simulink model "dimen"  (R2013a)
settings: Solver=ode23tb  StartTime=0.0  StopTime=10.0  RelTol=1e-4
values from neighbouring files (symbols this model uses):
  Cf = 1e-3    (= 0.001)    [dimensionamento.m]
  D0 = 50    [dimensionamento.m]
  DF = 100    [dimensionamento.m]
  ftr = 10e3    (= 10000)    [dimensionamento.m]
  J = 2.22e-2    (= 0.0222)    [dimensionamento.m]
  kt = kt1    [dimensionamento.m]
  La = 28e-3    (= 0.028)    [dimensionamento.m]
  Ra = 2.58    [dimensionamento.m]
  Vsource = Vnom    (= 240)    [dimensionamento.m]
libraries: powerlib x9, simulink x2
settings Model: Creator=dello  LastModifiedBy=dello
settings SolverCC: SolverResetMethod=Robust
settings DataIOCC: SignalLoggingSaveFormat=ModelDataLogs  SignalLoggingName=results

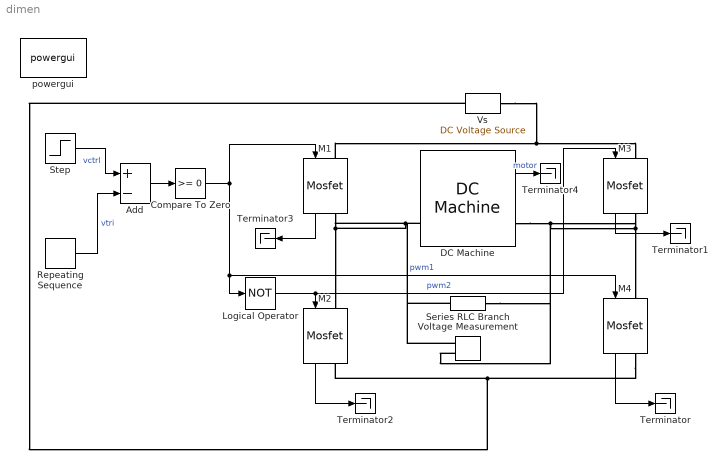
== system dimen ==
  Add : Sum  Inputs=+-
  Compare To Zero : simulink/Logic and Bit Operations/Compare To Zero  relop=>=  OutDataTypeStr=boolean
  DC Machine : powerlib/Machines/DC Machine  PresetModel=No  MechanicalLoad=Torque TL  FieldType=Permanent magnet  ShowDetailedParameters=on  RLa=[ Ra La]  RLf="[ 240  120]"  Laf=1.8  MachineConstant=Torque constant (N.m/A)  Ke=1.8  Kt=kt  J=J  Bm=B  Tf=0  w0=0  Ifinit=1  TsPowergui=0  TsBlock=-1
  Logical Operator : Logic  Operator=NOT  IconShape=distinctive  AllPortsSameDT=off  OutDataTypeStr=boolean
  M{1..4} (4 alike) : powerlib/Power Electronics/Mosfet  Ron=0.1  Lon=0  Rd=0.01  Vfd=0  IC=0  Rs=1e5  Cs=inf  Measurements=on
  Repeating Sequence : simulink/Sources/Repeating Sequence  rep_seq_t=[0 1/ftr/2 1/ftr]  rep_seq_y=[0 100 0]
  Series RLC Branch : powerlib/Elements/Series RLC Branch  LConnTagsString=__new0  RConnTagsString=__new0  BranchType=C  Resistance=1  Inductance=1e-3  SetiL0=off  InitialCurrent=0  Capacitance=Cf  Setx0=off  InitialVoltage=0  Measurements=None
  Step : Step  Before=D0  After=DF  SampleTime=0
  Terminator{,1..4} (5 alike) : Terminator
  Voltage Measurement : powerlib/Measurements/Voltage Measurement  PhasorSimulation=off  OutputType=Complex  PSBequivalent=0
  Vs : powerlib/Electrical Sources/DC Voltage Source  Amplitude=Vsource  Measurements=None
  powergui : powerlib/powergui  Priority=1  SimulationMode=Continuous  SolverType=Tustin  SampleTime=50e-6  frequency=60  SPID=off  DisableSnubberDevices=off  DisableRonSwitches=off  DisableVfSwitches=off  SwTol=0  Interpol=off  DisplayEquations=off  frequencyindice=0  Pbase=100e6  ErrMax=1e-4  Iterations=50  UnitsV=kV  UnitsW=MW  FunctionMessages=off  echomessages=off  HookPort=off  EnableUseOfTLC=off  x0status=blocks  RestoreLinks=warning  ResistiveCurrentMeasurement=off  Frange=[0:2:500]  Ylog=off  Xlog=on  ShowGrid=off  save=off  variable=ZData  ZoomFFT=off  StartTime=0.0  cycles=1  DisplayStyle=1  fundamental=60  FreqAxis=off  MaxFrequency=1000  frequencyindicesteady=1  RmsSteady=1  display=off  Ts=0  methode=off
  wires:
  Logical Operator/1 -> M2/1, M3/1  "pwm2"
  Compare To Zero/1 -> M1/1, M4/1, Logical Operator/1  "pwm1"
  Step/1 -> Add/1  "vctrl"
  Repeating Sequence/1 -> Add/2  "vtri"
  Add/1 -> Compare To Zero/1
  M4/1 -> Terminator/1
  M3/1 -> Terminator1/1
  M2/1 -> Terminator2/1
  M1/1 -> Terminator3/1
  DC Machine/1 -> Terminator4/1  "motor"
  connections:
  M3/RConn1 -- Series RLC Branch/RConn1 -- Voltage Measurement/LConn2 -- DC Machine/RConn1 -- M4/LConn1
  M1/RConn1 -- Series RLC Branch/LConn1 -- Voltage Measurement/LConn1 -- DC Machine/LConn1 -- M2/LConn1
  M1/LConn1 -- Vs/RConn1 -- M3/LConn1
  M4/RConn1 -- Vs/LConn1 -- M2/RConn1
